simulink model "sim06"  (R2012b)
settings: Solver=ode3  StartTime=0.0  StopTime=10.0  FixedStep=0.01  RelTol=1e-3
settings Model: Creator=Administrator  LastModifiedBy=Administrator

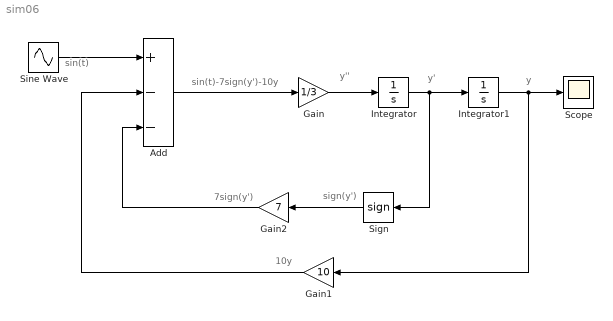
== system sim06 ==
  note: sin(t)
  note: sin(t)-7sign(y')-10y
  note: 10y
  note: 7sign(y')
  note: sign(y')
  note: y
  note: y'
  note: y''
  Add : Sum  Inputs=+--
  Gain : Gain  Gain=1/3
  Gain1 : Gain  Gain=10
  Gain2 : Gain  Gain=7
  Integrator : Integrator
  Integrator1 : Integrator  InitialCondition=5
  Scope : Scope
  Sign : Signum
  Sine Wave : Sin  SampleTime=0
  wires:
  Add/1 -> Gain/1
  Gain/1 -> Integrator/1
  Integrator/1 -> Sign/1, Integrator1/1
  Integrator1/1 -> Gain1/1, Scope/1
  Sine Wave/1 -> Add/1
  Sign/1 -> Gain2/1
  Gain1/1 -> Add/2
  Gain2/1 -> Add/3
